simulink model "BalanceMultiNew"  (Simulink 8.1)
settings: Solver=ode3  SolverMode=SingleTasking  StartTime=0.0  StopTime=10.0  RelTol=1e-3
PreLoadFcn:
  | waijung.modelPreload; % Required for working with Waijung Blockset. Do not remove.
undefined symbols (not defined in the file): ARM, DIR, disable_customio, enable_customio, in1, in2, inalpha, intheta, Link, LQFP100, MDK, out1, out2, output_customio, PD12, ST, STM32F407VG, STM32F4DISCOVERY
libraries: stm32f4_io_lib x2, fuzblock x2, waijung_customcode x1, stm32f4_device_config_lib x1
(part 2 of 2)

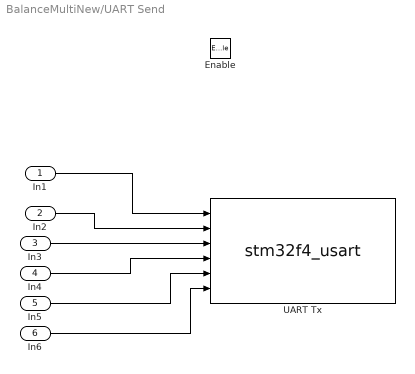
== system BalanceMultiNew/UART Send ==
  In1 : Inport
  In2 : Inport  Port=2
  In3 : Inport  Port=3
  In4 : Inport  Port=4
  In5 : Inport  Port=5
  In6 : Inport  Port=6
  Enable : EnablePort
  UART Tx : S-Function  Priority=1  FunctionName=stm32f4_usart  Parameters=configuration,uartmodule,transfer,baudrate,inputtype,outputtype,confstr,binheaderarray,binterminatorarray,asciiheader,asciiterminator,bindatalength,packetmode,varname,sampletime,sampletimestr,blockid  EnableBusSupport=off  mask(stm32f4_usart){configuration=Tx, uartmodule=1, baudrate=115200, databits=8, parity=No, stopbit=1, remaptxpin=Not used, remaprxpin=Not used, flowcontrol=None, remapctspin=Not used, remaprtspin=Not used, advanceoptions=off, rxbuffersize=512, txbuffersize=512, transfer=Blocking, packetmode=Ascii, binheader='7E 7E', binterminator='03 03', porttype_double=6, porttype_single=0, porttype_int8=0, porttype_uint8=0, porttype_int16=0, porttype_uint16=0, porttype_int32=0, porttype_uint32=0, asciiformat='a,%f,%f,%f,%f,%f,%f,', rx_asciiterminator=CRLF (0x0D 0x0A - "\r\n"), tx_asciiterminator=LF (0x0A - "\n"), storagename=<empty>, varname=, inputtype=[6  1 1 1 1 1 1], outputtype=[0], binheaderarray=[0], binterminatorarray=[0], bindatalength=0, asciiheader='a,%f,%f,%f,%f,%f,%f,\n', asciiterminator=[1 10], sampletime=-1, sampletimestr=0.01, blockid=UARTSendUARTTx, confstr=[ "dummy", "0", "*", "*", "0", "*", "*", "0", "*", "*", "0", "*", "*", "2", "4", "7", "2", "4", "2", "512", "512", "2", "1", "115200", "8", "No", "1", "None", "USART1"], lastmodule=1}
      mask prompts: uartmodule "UART Module"; baudrate "Baud rate (bps)"; databits "Data bits"; stopbit "Stop bit"; remaptxpin "Tx Pin"; remaprxpin "Rx Pin"; flowcontrol "Hardware flow control"; remapctspin "HW Flow control, CTS Pin"; remaprtspin "HW Flow control, RTS Pin"; advanceoptions "Advance options"; rxbuffersize "Rx buffer size (bytes)"; txbuffersize "Tx buffer size (bytes)"; packetmode "Packet mode"; binheader "Binary header (example: '7E 7E')"; binterminator "Binary terminator (example: '03 03')"; porttype_double "Number of data port, type DOUBLE"; porttype_single "Number of data port, type SINGLE"; porttype_int8 "Number of data port, type INT8"; porttype_uint8 "Number of data port, type UINT8"; porttype_int16 "Number of data port, type INT16"; porttype_uint16 "Number of data port, type UINT16"; porttype_int32 "Number of data port, type INT32"; porttype_uint32 "Number of data port, type UINT32"; asciiformat "Ascii format"; rx_asciiterminator "End of packet"; tx_asciiterminator "End of packet"; storagename "Buffer"; varname "Var name"; inputtype "Input data type"; outputtype "Output data type"; binheaderarray "Binary header"; binterminatorarray "Binary terminator"; bindatalength "Binary data length"; asciiheader "Ascii header (printf format)"; asciiterminator "Ascii terminator"; sampletime "Sample time (sec)"; sampletimestr "Compiled sample time (sec) in string"; confstr "Configuration string"; lastmodule "Last module selected"
      mask help:
      | Data type for Ascii format
      | %u, %i, %d, %o, %x: uint32
      | %e, %g, %f: single
      | %c: int8
      mask init:
      | stm32f4_usart_callback('init');
      mask Help: web(fullfile(waijungdocroot,'stm32f4_usart_tx.htm'), '-browser')
      mask TypeOptions configuration: Setup | Tx | Rx
      mask Callback configuration: stm32f4_usart_callback('configuration');
      mask TypeOptions uartmodule: 1 | 2 | 3 | 4 | 5 | 6
      mask Callback uartmodule: stm32f4_usart_callback('uartmodule');
      mask Callback baudrate: stm32f4_usart_callback('baudrate');
      mask TypeOptions databits: 8
      mask TypeOptions parity: No | Odd | Even
      mask TypeOptions stopbit: 0.5 | 1 | 1.5 | 2
      mask TypeOptions remaptxpin: Not used | A9 | B6
      mask TypeOptions remaprxpin: Not used | A10 | B7
      mask TypeOptions flowcontrol: None | RTS | CTS | RTS/CTS
      mask Callback flowcontrol: stm32f4_usart_callback('flowcontrol');
      mask TypeOptions remapctspin: Not used | A11
      mask TypeOptions remaprtspin: Not used | A12
      mask Callback advanceoptions: stm32f4_usart_callback('advanceoptions');
      mask TypeOptions rxbuffersize: 16 | 32 | 64 | 128 | 256 | 512 | 1024 | 2048
      mask TypeOptions txbuffersize: 16 | 32 | 64 | 128 | 256 | 512 | 1024 | 2048
      mask TypeOptions transfer: Blocking | Non-Blocking
      mask Callback transfer: stm32f4_usart_callback('transfer');
      mask TypeOptions packetmode: Ascii | Binary | String Buffer
      mask Callback packetmode: stm32f4_usart_callback('packetmode');
      mask Callback binheader: stm32f4_usart_callback('binheader');
      mask Callback binterminator: stm32f4_usart_callback('binterminator');
      mask Callback porttype_double: stm32f4_usart_callback('porttype');
      mask Callback porttype_single: stm32f4_usart_callback('porttype');
      mask Callback porttype_int8: stm32f4_usart_callback('porttype');
      mask Callback porttype_uint8: stm32f4_usart_callback('porttype');
      mask Callback porttype_int16: stm32f4_usart_callback('porttype');
      mask Callback porttype_uint16: stm32f4_usart_callback('porttype');
      mask Callback porttype_int32: stm32f4_usart_callback('porttype');
      mask Callback porttype_uint32: stm32f4_usart_callback('porttype');
      mask Callback asciiformat: stm32f4_usart_callback('asciiformat');
      mask TypeOptions rx_asciiterminator: CR (0x0D - "\r") | LF (0x0A - "\n") | CRLF (0x0D 0x0A - "\r\n")
      mask Callback rx_asciiterminator: stm32f4_usart_callback('rx_asciiterminator');
      mask TypeOptions tx_asciiterminator: CR (0x0D - "\r") | LF (0x0A - "\n") | CRLF (0x0D 0x0A - "\r\n") | None
      mask Callback tx_asciiterminator: stm32f4_usart_callback('tx_asciiterminator');
      mask TypeOptions storagename: <empty>
      mask Callback storagename: stm32f4_usart_callback('storagename');
      mask Callback varname: stm32f4_usart_callback('varname');
      mask Callback sampletime: stm32f4_usart_callback('sampletime');
      mask Callback sampletimestr: stm32f4_usart_callback('sampletimestr');
      mask Callback blockid: stm32f4_usart_callback('blockid');
      mask Display: text(0.95, 0.5, 'Module: USART1_Tx\nPacket: Ascii\nTransfer: Blocking\nTs (sec): 0.01','ver','middle','hor','right'); port_label('input', 1,'single'); port_label('input', 2,'single'); port_label('input', 3,'single'); port_label('input', 4,'single'); port_label('input', 5,'single'); port_label('input', 6,'single');
  wires:
  In1/1 -> UART Tx/1
  In2/1 -> UART Tx/2
  In3/1 -> UART Tx/3
  In4/1 -> UART Tx/4
  In5/1 -> UART Tx/5
  In6/1 -> UART Tx/6

== matlab function V_control ==
  data: u input double; PWM output double; DIR output double
function [PWM, DIR] = fcn(u)
%#codegen
if u<0
    DIR=0;
    PWM=-u*100/24;
else
%     DIR=1;
%     PWM=u*100/24;
DIR=1;
PWM=u*100/24;

end

== matlab function Subsystem/EnergySWINGUP ==
  data: u output double; alpha input double; alphadot input double
%#************************
%energy based control
%#***********************88

function u = SWING_UP(alpha,alphadot)
%if (alpha>0.6)||(alpha<-0.6)
voltage=3.5;
if (alphadot*cos(alpha))<0
    u=-voltage;
% % % % % % elseif (alphadot*cos(alpha))>0
% % % % % %     u=voltage;
% if(q1>pi)&&(q1<2*pi)
%     q1=q1-2*pi;
% if(abs(q2)<pi/2)
% if((alpha>=pi)&&(alpha<3*pi/2)&&(alphadot<=0))
%     u=20;
% elseif ((alpha<pi)&&(alpha>pi/2)&&(alphadot>0))
%     u=-20;
% % if((alpha>=-pi)&&(alpha<-pi/2)&&(alphadot<=0))
% %     u=10;
% % elseif ((alpha<pi)&&(alpha>pi/2)&&(alphadot>0))
% %     u=-10;
% elseif ((abs(q1)< pi/18))
%     u = -(q2*(-10)+ q1*(53.5434) + q2dot*(-4.9882) + q1dot*(7.4922));
% else
%     u = 0;
% end
% elseif(q2>pi)
%     u=-3;
else
    u=voltage;
end
%else u=0;
end



% if u >=24
%     u = 24;
% end
% if u <= -24
%     u = -24;
% end -10.0000   53.5434   -4.9882    7.4922

== matlab function Switch_Funciton ==
  data: alpha input double; sw output double
function sw = Switch(alpha)
if (alpha<0.5)&&(alpha>-0.5)
    sw = 0;
else
    sw = 1;
end

== matlab function MATLAB Function ==
  data: x output double; a input double; y output double; b input double; c input double
function[x,y] = fcn(a, b, c)
%#codegen
if(a==true)
    x=b;
    y=c;
else
    x=0;y=0;
end

== matlab function Multi_Controllers/MATLAB Function ==
  data: option input double; Vcontrol output double; lqr input double; fuzzysingle input double; fuzzy input double
function Vcontrol = Choose(option, lqr, fuzzysingle, fuzzy)
%#codegen
if(option==0)
    Vcontrol=lqr;
elseif(option==1)
    Vcontrol=fuzzysingle;
else Vcontrol=fuzzy;
end

== matlab function Subsystem/SWINGUP ==
  data: u output double; alpha input double; alphadot input double
%#************************
%energy based control
%#***********************88

function u = SWING_UP(alpha,alphadot)
%if (alpha>0.6)||(alpha<-0.6)
voltage=7.5;
% if (alphadot*cos(alpha))<0
%     u=-voltage;
% % % % % % elseif (alphadot*cos(alpha))>0
% % % % % %     u=voltage;
% if(q1>pi)&&(q1<2*pi)
%     q1=q1-2*pi;
% if(abs(q2)<pi/2)
% if((alpha>=pi)&&(alpha<3*pi/2)&&(alphadot<=0))
%     u=20;
% elseif ((alpha<pi)&&(alpha>pi/2)&&(alphadot>0))
%     u=-20;
if((alpha>=-pi)&&(alpha<-pi/2)&&(alphadot<=0))
    u=voltage;
elseif ((alpha<pi)&&(alpha>pi/2)&&(alphadot>0))
    u=-voltage;
% elseif ((abs(q1)< pi/18))
%     u = -(q2*(-10)+ q1*(53.5434) + q2dot*(-4.9882) + q1dot*(7.4922));
% else
%     u = 0;
% end
% elseif(q2>pi)
%     u=-3;
else
    u=0;
end
%else u=0;
%end



% if u >=24
%     u = 24;
% end
% if u <= -24
%     u = -24;
% end -10.0000   53.5434   -4.9882    7.4922

== matlab function Subsystem/Choose_Swing ==
  data: sw input double; Swing output double; energy input double; errSwing input double; energyLQR input double
function Swing = Choose(sw,energy,errSwing,energyLQR)
%#codegen

if(sw==0)
    Swing=energy;
elseif(sw==1)
        Swing=errSwing;
    else Swing=energyLQR;
     
end

== matlab function Subsystem/EnergySWINGUP1 ==
  data: u output double; alpha input double; alphadot input double
%#************************
%energy based control
%#***********************88

function u = SWING_UP(alpha,alphadot)
%if (alpha>0.6)||(alpha<-0.6)
voltage=5;
if (alphadot*cos(alpha))<0
    u=-voltage;
% % % % % % elseif (alphadot*cos(alpha))>0
% % % % % %     u=voltage;
% if(q1>pi)&&(q1<2*pi)
%     q1=q1-2*pi;
% if(abs(q2)<pi/2)
% if((alpha>=pi)&&(alpha<3*pi/2)&&(alphadot<=0))
%     u=20;
% elseif ((alpha<pi)&&(alpha>pi/2)&&(alphadot>0))
%     u=-20;
% % if((alpha>=-pi)&&(alpha<-pi/2)&&(alphadot<=0))
% %     u=10;
% % elseif ((alpha<pi)&&(alpha>pi/2)&&(alphadot>0))
% %     u=-10;
% elseif ((abs(q1)< pi/18))
%     u = -(q2*(-10)+ q1*(53.5434) + q2dot*(-4.9882) + q1dot*(7.4922));
% else
%     u = 0;
% end
% elseif(q2>pi)
%     u=-3;
else
    u=voltage;
end
%else u=0;
end



% if u >=24
%     u = 24;
% end
% if u <= -24
%     u = -24;
% end -10.0000   53.5434   -4.9882    7.4922

== matlab function Encoders/MATLAB Function ==
  data: pulsealpha input double; alphadisplay output double; alpha output double
function [alphadisplay,alpha] = alpha_pulse(pulsealpha)
%#codegen
alphadisplay=pulsealpha*2*pi/4096+pi;
alpha =mod((alphadisplay-pi),(2*pi))-pi;

== matlab function Encoders/MATLAB Function1 ==
  data: pulsetheta input double; thetadisplay output double; theta output double
function [thetadisplay,theta] = theta_pulse(pulsetheta)
%#codegen
thetadisplay=pulsetheta*2*pi/4000;
theta=mod((thetadisplay+pi),(2*pi))-pi;

== matlab function Multi_Controllers/MATLAB Function1 ==
  data: alpha input double; y output double; alphadot input double; theta input double; thetadot input double
function y = convert(alpha, alphadot,theta,thetadot)
%#codegen
lamda1=1;
lamda2=1;
lamda3=1;
y = (alpha+alphadot*lamda1+theta*lamda2+thetadot*lamda3)/sqrt(1+lamda1*lamda1+lamda2*lamda2+lamda3*lamda3);
